simulink model "ex1"  (R2018b)
settings: Solver=VariableStepAuto  StartTime=0.0  StopTime=10.0  RelTol=1e-3
settings Model: host=localhost  port=6379  Creator=valber  LastModifiedBy=valber

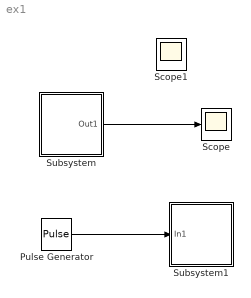
== system ex1 ==
  Pulse Generator : DiscretePulseGenerator  Amplitude=10
  Scope : Scope
  Subsystem : Subsystem  mask{host=localhost, port=6379, key=key}
      mask prompts: host "Redis hostname"; port "Redis port"; key "Probing key"
  Subsystem1 : Subsystem  mask{host=localhost, port=6379, key=key}
  Scope1 : Scope
  wires:
  Subsystem/1(Out1) -> Scope/1
  Pulse Generator/1 -> Subsystem1/1(In1)

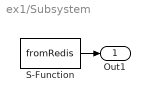
== system ex1/Subsystem ==
  S-Function : S-Function  FunctionName=fromRedis  Parameters=host, port, key  SFunctionDeploymentMode=off  EnableBusSupport=off
  Out1 : Outport
  wires:
  S-Function/1 -> Out1/1

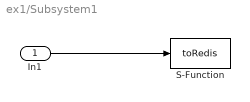
== system ex1/Subsystem1 ==
  In1 : Inport
  S-Function : S-Function  FunctionName=toRedis  Parameters=host,port,key  SFunctionDeploymentMode=off  EnableBusSupport=off
  wires:
  In1/1 -> S-Function/1
